simulink model "ModeleRobot"  (Simulink 7.4)
settings: Solver=FixedStepDiscrete  StartTime=0.0  StopTime=Inf  FixedStep=Te  RelTol=1e-3
libraries: simulink x10
CloseFcn:
  | rtwprivate ssgencode ModelCloseRequest ModeleRobot
settings Model: Creator=Admin  LastModifiedBy=Admin
settings DataIOCC: LimitDataPoints=off  SaveFormat=StructureWithTime
settings OptimizationCC: UseIntDivNetSlope=on  PassReuseOutputArgsAs=Individual arguments  ZeroExternalMemoryAtStartup=off  ZeroInternalMemoryAtStartup=off  EfficientFloat2IntCast=on  OptimizeModelRefInitCode=on  LifeSpan=Inf
settings DebuggingCC: SaveWithParameterizedLinksMsg=none  SignalResolutionControl=TryResolveAllWithWarning  MultiTaskDSMMsg=warning  MultiTaskCondExecSysMsg=none
settings HardwareCC: ProdIntDivRoundTo=Zero  ProdEndianess=LittleEndian  ProdHWDeviceType=Generic->32-bit x86 compatible
settings SFSimCC: SFSimEnableDebug=off  SFSimOverflowDetection=off  SFSimEcho=off  SimIntegrity=off  SimBuildMode=sf_nonincremental_build
settings RTWCC: SystemTargetFile=ert.tlc  GenCodeOnly=on  GenerateMakefile=off  TemplateMakefile=ert_default_tmf  PostCodeGenCommand=packNGo(buildInfo);  Description=Real-Time Workshop Embedded Coder  ProcessScript=ert_make_rtw_hook  IncludeERTFirstTime=on  RTWCompilerOptimization=On  CheckMdlBeforeBuild=Warning
settings CodeAppCC: IgnoreCustomStorageClasses=off
settings ERTTargetCC: UtilityFuncGeneration=Shared location  MultiwordLength=2048  IncludeMdlTerminateFcn=off  SuppressErrorStatus=on  SupportNonFinite=off  ERTCustomFileTemplate=example_file_process.tlc  GlobalDataDefinition=InSourceFile  GlobalDataReference=InSourceFile  ConvertIfToSwitch=off

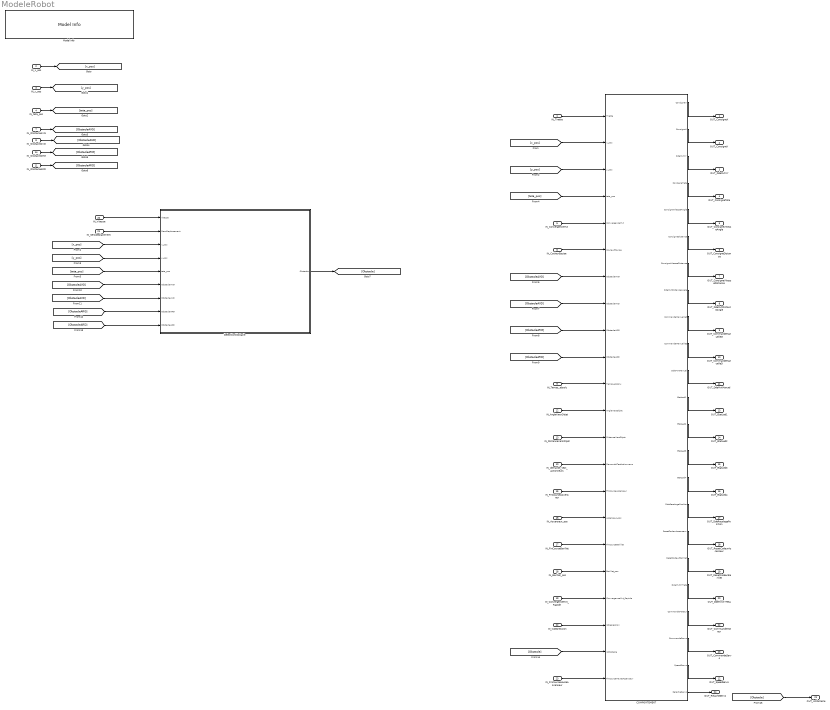
== system ModeleRobot ==
  IN_Tirette : Inport  OutDataType=sfix(16)  OutScaling=2^0
  IN_x_pos : Inport  Port=2  OutDataType=sfix(16)  OutScaling=2^0
  IN_y_pos : Inport  Port=3  OutDataType=sfix(16)  OutScaling=2^0
  IN_teta_pos : Inport  Port=4  OutDataType=sfix(16)  OutScaling=2^0
  IN_ConvergenceMvt : Inport  Port=5  OutDataType=sfix(16)  OutScaling=2^0
  IN_CouleurEquipe : Inport  Port=6  OutDataType=sfix(16)  OutScaling=2^0
  IN_ObstacleAVG : Inport  Port=7  OutDataType=sfix(16)  OutScaling=2^0
  IN_ObstacleAVD : Inport  Port=8  OutDataType=sfix(16)  OutScaling=2^0
  IN_Temps_absolu : Inport  Port=9  OutDataType=sfix(16)  OutScaling=2^0
  IN_demande_test_actionneurs : Inport  Port=10  OutDataType=sfix(16)  OutScaling=2^0
  IN_ObstacleARD : Inport  Port=11  OutDataType=sfix(16)  OutScaling=2^0
  IN_AngleVersObjet : Inport  Port=12  OutDataType=sfix(16)  OutScaling=2^0
  IN_DistanceVersObjet : Inport  Port=13  OutDataType=sfix(16)  OutScaling=2^0
  IN_ObstacleARG : Inport  Port=14  OutDataType=sfix(16)  OutScaling=2^0
  IN_FinCourseAscenseur : Inport  Port=15  OutDataType=sfix(16)  OutScaling=2^0
  IN_Ascenseur_pos : Inport  Port=16  OutDataType=sfix(16)  OutScaling=2^0
  IN_FinCourseBarillet : Inport  Port=17  OutDataType=sfix(16)  OutScaling=2^0
  IN_Barillet_pos : Inport  Port=18  OutDataType=sfix(16)  OutScaling=2^0
  IN_ConvergenceMvt_Rapide : Inport  Port=19  OutDataType=sfix(16)  OutScaling=2^0
  IN_Vitesse : Inport  Port=20  OutDataType=sfix(16)  OutScaling=2^0
  IN_SensDeplacement : Inport  Port=21  OutDataType=sfix(16)  OutScaling=2^0
  IN_isDepression : Inport  Port=22  OutDataType=sfix(16)  OutScaling=2^0
  IN_FinCourseHauteAscenseur : Inport  Port=23  OutDataType=sfix(16)  OutScaling=2^0
  COMPORTEMENT : Stateflow chart
  DetectionObstacle : Subsystem
  Model Info : simulink/Model-Wide Utilities/Model Info  SystemSampleTime=-1  InitialBlockCM=None  BlockCM=None  Frame=on  DisplayStringWithTags=|  HorizontalTextAlignment=Left  LeftAlignmentValue=0.02  SourceBlockDiagram=ModeleRobot  TagMaxNumber=20
      | Description du comportement d'un robot
      | Objectif du robot :
  OUT_ConsigneX : Outport  OutDataType=sfix(16)  OutScaling=2^0
  OUT_ConsigneY : Outport  Port=2  OutDataType=sfix(16)  OutScaling=2^0
  OUT_DdeMvtXY : Outport  Port=3  OutDataType=sfix(16)  OutScaling=2^0
  OUT_ConsigneTeta : Outport  Port=4  OutDataType=sfix(16)  OutScaling=2^0
  OUT_ConsigneVitesseAngle : Outport  Port=5  OutDataType=sfix(16)  OutScaling=2^0
  OUT_ConsigneDistance : Outport  Port=6  OutDataType=sfix(16)  OutScaling=2^0
  OUT_ConsigneVitesseDistance : Outport  Port=7  OutDataType=sfix(16)  OutScaling=2^0
  OUT_DdeMvtDistanceAngle : Outport  Port=8  OutDataType=sfix(16)  OutScaling=2^0
  OUT_CommandeManuelleG : Outport  Port=9  OutDataType=sfix(16)  OutScaling=2^0
  OUT_CommandeManuelleD : Outport  Port=10  OutDataType=sfix(16)  OutScaling=2^0
  OUT_DdeMvtManuel : Outport  Port=11  OutDataType=sfix(16)  OutScaling=2^0
  OUT_SpeedServo : Outport  Port=12  OutDataType=sfix(16)  OutScaling=2^0
  OUT_EtatLed1 : Outport  Port=13  OutDataType=sfix(16)  OutScaling=2^0
  OUT_EtatLed2 : Outport  Port=14  OutDataType=sfix(16)  OutScaling=2^0
  OUT_EtatLed3 : Outport  Port=15  OutDataType=sfix(16)  OutScaling=2^0
  OUT_EtatLed4 : Outport  Port=16  OutDataType=sfix(16)  OutScaling=2^0
  OUT_DdeRecalagePosition : Outport  Port=17  OutDataType=sfix(16)  OutScaling=2^0
  OUT_ResetCodeurAscenseur : Outport  Port=18  OutDataType=sfix(16)  OutScaling=2^0
  OUT_ResetCodeurBarillet : Outport  Port=19  OutDataType=sfix(16)  OutScaling=2^0
  OUT_DdeMvtXYTeta : Outport  Port=20  OutDataType=sfix(16)  OutScaling=2^0
  OUT_isObstacle : Outport  Port=21  OutDataType=sfix(16)  OutScaling=2^0
  OUT_CommandeMoteur : Outport  Port=22  OutDataType=sfix(16)  OutScaling=2^0
  OUT_CommandeServo : Outport  Port=23  OutDataType=sfix(16)  OutScaling=2^0
  OUT_RelacheServo : Outport  Port=24  OutDataType=sfix(16)  OutScaling=2^0
  wires:
  COMPORTEMENT/1(ConsigneX) -> OUT_ConsigneX/1
  COMPORTEMENT/2(ConsigneY) -> OUT_ConsigneY/1
  IN_Temps_absolu/1 -> COMPORTEMENT/11(Temps_absolu)
  IN_ConvergenceMvt/1 -> COMPORTEMENT/5(ConvergenceMvt)
  IN_CouleurEquipe/1 -> COMPORTEMENT/6(CouleurEquipe)
  IN_Tirette/1 -> COMPORTEMENT/1(Tirette)
  IN_demande_test_actionneurs/1 -> COMPORTEMENT/14(DemandeTestActionneurs)
  IN_AngleVersObjet/1 -> COMPORTEMENT/12(AngleVersObjet)
  IN_DistanceVersObjet/1 -> COMPORTEMENT/13(DistanceVersObjet)
  COMPORTEMENT/3(DdeMvtXY) -> OUT_DdeMvtXY/1
  COMPORTEMENT/4(ConsigneTeta) -> OUT_ConsigneTeta/1
  COMPORTEMENT/5(ConsigneVitesseAngle) -> OUT_ConsigneVitesseAngle/1
  COMPORTEMENT/6(ConsigneDistance) -> OUT_ConsigneDistance/1
  COMPORTEMENT/7(ConsigneVitesseDistance) -> OUT_ConsigneVitesseDistance/1
  COMPORTEMENT/8(DdeMvtDistanceAngle) -> OUT_DdeMvtDistanceAngle/1
  COMPORTEMENT/9(CommandeManuelleG) -> OUT_CommandeManuelleG/1
  COMPORTEMENT/10(CommandeManuelleD) -> OUT_CommandeManuelleD/1
  COMPORTEMENT/11(DdeMvtManuel) -> OUT_DdeMvtManuel/1
  COMPORTEMENT/22(SpeedServo) -> OUT_SpeedServo/1
  COMPORTEMENT/12(EtatLed1) -> OUT_EtatLed1/1
  COMPORTEMENT/13(EtatLed2) -> OUT_EtatLed2/1
  COMPORTEMENT/14(EtatLed3) -> OUT_EtatLed3/1
  COMPORTEMENT/15(EtatLed4) -> OUT_EtatLed4/1
  COMPORTEMENT/16(DdeRecalagePosition) -> OUT_DdeRecalagePosition/1
  COMPORTEMENT/17(ResetCodeurAscenseur) -> OUT_ResetCodeurAscenseur/1
  COMPORTEMENT/18(ResetCodeurBarillet) -> OUT_ResetCodeurBarillet/1
  [x_pos] -> COMPORTEMENT/2(x_pos)
  [y_pos] -> COMPORTEMENT/3(y_pos)
  [teta_pos] -> COMPORTEMENT/4(teta_pos)
  IN_Vitesse/1 -> DetectionObstacle/1(Vitesse)
  IN_SensDeplacement/1 -> DetectionObstacle/2(SensDeplacement)
  [x_pos] -> DetectionObstacle/3(x_pos)
  [y_pos] -> DetectionObstacle/4(y_pos)
  [teta_pos] -> DetectionObstacle/5(teta_pos)
  IN_x_pos/1 -> [x_pos]
  IN_y_pos/1 -> [y_pos]
  IN_teta_pos/1 -> [teta_pos]
  COMPORTEMENT/19(DdeMvtXYTeta) -> OUT_DdeMvtXYTeta/1
  IN_ObstacleAVG/1 -> [ObstacleAVG]
  IN_ObstacleAVD/1 -> [ObstacleAVD]
  IN_ObstacleARG/1 -> [ObstacleARG]
  IN_ObstacleARD/1 -> [ObstacleARD]
  [ObstacleAVG] -> COMPORTEMENT/7(ObstacleAVG)
  [ObstacleAVD] -> COMPORTEMENT/8(ObstacleAVD)
  [ObstacleARG] -> COMPORTEMENT/9(ObstacleARG)
  [ObstacleARD] -> COMPORTEMENT/10(ObstacleARD)
  [ObstacleAVG] -> DetectionObstacle/6(ObstacleAVG)
  [ObstacleAVD] -> DetectionObstacle/7(ObstacleAVD)
  [ObstacleARG] -> DetectionObstacle/8(ObstacleARG)
  [ObstacleARD] -> DetectionObstacle/9(ObstacleARD)
  DetectionObstacle/1(Obstacle) -> [Obstacle]
  IN_FinCourseAscenseur/1 -> COMPORTEMENT/15(FinCourseAscenseur)
  [Obstacle] -> COMPORTEMENT/21(isObstacle)
  IN_FinCourseHauteAscenseur/1 -> COMPORTEMENT/22(FinCourseHauteAscenseur)
  IN_Ascenseur_pos/1 -> COMPORTEMENT/16(Ascenseur_pos)
  IN_FinCourseBarillet/1 -> COMPORTEMENT/17(FinCourseBarillet)
  IN_Barillet_pos/1 -> COMPORTEMENT/18(Barillet_pos)
  IN_ConvergenceMvt_Rapide/1 -> COMPORTEMENT/19(ConvergenceMvt_Rapide)
  IN_isDepression/1 -> COMPORTEMENT/20(isDepression)
  [Obstacle] -> OUT_isObstacle/1
  COMPORTEMENT/21(CommandeServo) -> OUT_CommandeServo/1
  COMPORTEMENT/20(CommandeMoteur) -> OUT_CommandeMoteur/1
  COMPORTEMENT/23(RelacheServo) -> OUT_RelacheServo/1

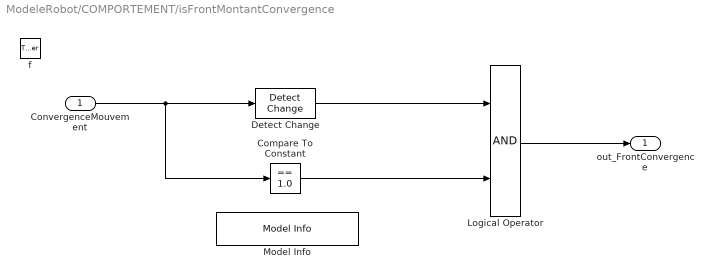
== system ModeleRobot/COMPORTEMENT/isFrontMontantConvergence ==
  ConvergenceMouvement : Inport
  f : TriggerPort  TriggerType=function-call
      settings: CopyFcn=set_param(gcbh,'PreDeleteFcn','')  PreDeleteFcn=Stateflow.SLINSF.SimulinkMan.unsafePredeleteFcn
  Compare To Constant : simulink/Logic and Bit Operations/Compare To Constant  SystemSampleTime=-1  relop===  const=1.0  LogicOutDataTypeMode=uint8
  Detect Change : simulink/Logic and Bit Operations/Detect Change  SystemSampleTime=-1  vinit=0
  Logical Operator : Logic  AllPortsSameDT=off  OutDataTypeMode=boolean  LogicDataType=fixdt(0, 8)  OutDataTypeStr=boolean
  Model Info : simulink/Model-Wide Utilities/Model Info  SystemSampleTime=-1  InitialBlockCM=None  BlockCM=None  Frame=off  DisplayStringWithTags="\"1\" = mouvement terminé"  HorizontalTextAlignment=Center  LeftAlignmentValue=0.5  SourceBlockDiagram=ModeleRobot  TagMaxNumber=20
  out_FrontConvergence : Outport
  wires:
  ConvergenceMouvement/1 -> Detect Change/1, Compare To Constant/1
  Detect Change/1 -> Logical Operator/1
  Compare To Constant/1 -> Logical Operator/2
  Logical Operator/1 -> out_FrontConvergence/1

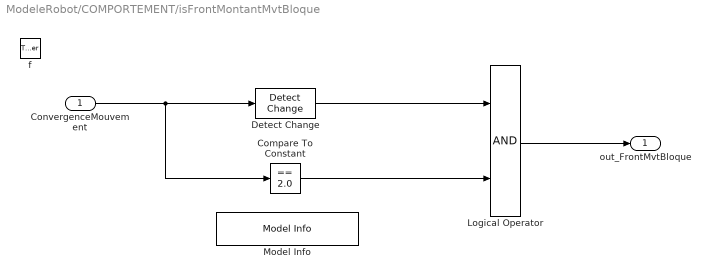
== system ModeleRobot/COMPORTEMENT/isFrontMontantMvtBloque ==
  ConvergenceMouvement : Inport
  f : TriggerPort  TriggerType=function-call
      settings: CopyFcn=set_param(gcbh,'PreDeleteFcn','')  PreDeleteFcn=Stateflow.SLINSF.SimulinkMan.unsafePredeleteFcn
  Compare To Constant : simulink/Logic and Bit Operations/Compare To Constant  SystemSampleTime=-1  relop===  const=2.0  LogicOutDataTypeMode=uint8
  Detect Change : simulink/Logic and Bit Operations/Detect Change  SystemSampleTime=-1  vinit=0
  Logical Operator : Logic  AllPortsSameDT=off  OutDataTypeMode=boolean  LogicDataType=fixdt(0, 8)  OutDataTypeStr=boolean
  Model Info : simulink/Model-Wide Utilities/Model Info  SystemSampleTime=-1  InitialBlockCM=None  BlockCM=None  Frame=off  DisplayStringWithTags="\"2\" = mouvement bloqué"  HorizontalTextAlignment=Center  LeftAlignmentValue=0.5  SourceBlockDiagram=ModeleRobot  TagMaxNumber=20
  out_FrontMvtBloque : Outport
  wires:
  ConvergenceMouvement/1 -> Detect Change/1, Compare To Constant/1
  Detect Change/1 -> Logical Operator/1
  Compare To Constant/1 -> Logical Operator/2
  Logical Operator/1 -> out_FrontMvtBloque/1

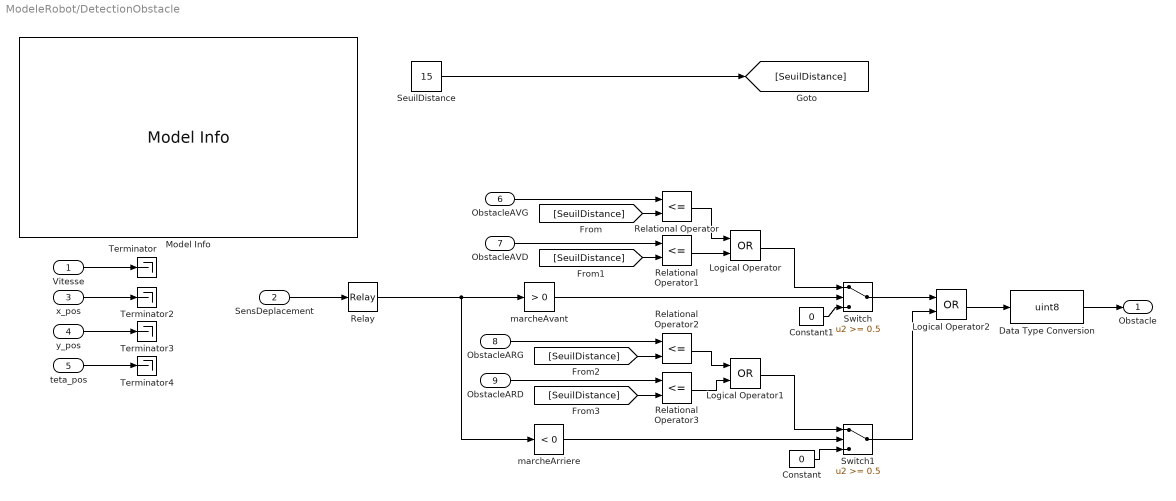
== system ModeleRobot/DetectionObstacle ==
  Vitesse : Inport  OutDataType=fixdt(1, 16)  OutScaling=2^0
  SensDeplacement : Inport  Port=2  OutDataType=fixdt(1, 16)  OutScaling=2^0
  x_pos : Inport  Port=3  OutDataType=fixdt(1, 16)  OutScaling=2^0
  y_pos : Inport  Port=4  OutDataType=fixdt(1, 16)  OutScaling=2^0
  teta_pos : Inport  Port=5  OutDataType=fixdt(1, 16)  OutScaling=2^0
  ObstacleAVG : Inport  Port=6  OutDataType=fixdt(1, 16)  OutScaling=2^0
  ObstacleAVD : Inport  Port=7  OutDataType=fixdt(1, 16)  OutScaling=2^0
  ObstacleARG : Inport  Port=8  OutDataType=fixdt(1, 16)  OutScaling=2^0
  ObstacleARD : Inport  Port=9  OutDataType=fixdt(1, 16)  OutScaling=2^0
  Constant : Constant  Value=0  OutDataType=fixdt(1, 16)  OutScaling=2^0
  Constant1 : Constant  Value=0  OutDataType=fixdt(1, 16)  OutScaling=2^0
  Data Type Conversion : DataTypeConversion  OutDataTypeMode=uint8  OutDataType=fixdt(1, 16)  OutScaling=2^0  OutDataTypeStr=uint8
  Logical Operator : Logic  Operator=OR  AllPortsSameDT=off  OutDataTypeMode=boolean  LogicDataType=fixdt(0, 8)  OutDataTypeStr=boolean
  Logical Operator1 : Logic  Operator=OR  AllPortsSameDT=off  OutDataTypeMode=boolean  LogicDataType=fixdt(0, 8)  OutDataTypeStr=boolean
  Logical Operator2 : Logic  Operator=OR  AllPortsSameDT=off  OutDataTypeMode=boolean  LogicDataType=fixdt(0, 8)  OutDataTypeStr=boolean
  Model Info : simulink/Model-Wide Utilities/Model Info  SystemSampleTime=-1  InitialBlockCM=None  BlockCM=None  Frame=on  DisplayStringWithTags=|  HorizontalTextAlignment=Left  LeftAlignmentValue=0.02  SourceBlockDiagram=ModeleRobot  TagMaxNumber=20
      | Description de la détection d'obstacle
      | Obstacle :
      | Suivant le sens de la marche on active la détection par capteur US (donne une distance). Fonction d'un seuil de distance on tilte sur la présence d'un obstacle. On synthétise les détection arrière et avant pour avoir une seule info de détection d'obstacle pour la stratégie.
      | 
      | TODO:
      | * faire varier le seuil de détection en fonction de la vitesse.
      | * utiliser la position et l'orientation du robot pour discriminer un élément du terrain.
  Relational Operator{,1..3} (4 alike) : RelationalOperator  Operator=<=  LogicOutDataTypeMode=boolean  LogicDataType=fixdt(0, 8)  OutDataTypeStr=boolean
  Relay : Relay  OnSwitchValue=1  OffSwitchValue=-1  OffOutputValue=-1  OutDataType=fixdt(1, 16)  OutScaling=2^0
  SeuilDistance : Constant  Value=15  OutDataType=fixdt(1, 16)  OutScaling=2^0
  Switch : Switch  Threshold=0.5  OutDataType=fixdt(1, 16)  OutScaling=2^0
  Switch1 : Switch  Threshold=0.5  OutDataType=fixdt(1, 16)  OutScaling=2^0
  Terminator{,2..4} (4 alike) : Terminator
  marcheArriere : simulink/Logic and Bit Operations/Compare To Zero  SystemSampleTime=-1  relop=<  LogicOutDataTypeMode=uint8
  marcheAvant : simulink/Logic and Bit Operations/Compare To Zero  SystemSampleTime=-1  relop=>  LogicOutDataTypeMode=uint8
  Obstacle : Outport  OutDataType=fixdt(1, 16)  OutScaling=2^0
  wires:
  Vitesse/1 -> Terminator/1
  SensDeplacement/1 -> Relay/1
  x_pos/1 -> Terminator2/1
  y_pos/1 -> Terminator3/1
  teta_pos/1 -> Terminator4/1
  marcheAvant/1 -> Switch/2
  Relational Operator1/1 -> Logical Operator/2
  ObstacleARD/1 -> Relational Operator3/1
  marcheArriere/1 -> Switch1/2
  Relational Operator2/1 -> Logical Operator1/1
  Constant/1 -> Switch1/3
  Switch/1 -> Logical Operator2/1
  Switch1/1 -> Logical Operator2/2
  Logical Operator2/1 -> Data Type Conversion/1
  Relational Operator/1 -> Logical Operator/1
  ObstacleAVG/1 -> Relational Operator/1
  ObstacleAVD/1 -> Relational Operator1/1
  ObstacleARG/1 -> Relational Operator2/1
  SeuilDistance/1 -> [SeuilDistance]
  [SeuilDistance] -> Relational Operator/2
  [SeuilDistance] -> Relational Operator3/2
  [SeuilDistance] -> Relational Operator2/2
  [SeuilDistance] -> Relational Operator1/2
  Constant1/1 -> Switch/3
  Relational Operator3/1 -> Logical Operator1/2
  Logical Operator1/1 -> Switch1/1
  Logical Operator/1 -> Switch/1
  Data Type Conversion/1 -> Obstacle/1
  Relay/1 -> marcheAvant/1, marcheArriere/1

== stateflow chart COMPORTEMENT ==
  state COMPORTEMENT_ROBOT [parallel]
    settings: executionOrder=1
    state ATTENTE_TIRETTE/
      state ACTIONNEURS_REPOS/ [parallel]
        settings: executionOrder=1
        state REPOS_SERVOS/
          entry :
          //on ne bouge pas en attendant le depart
          Mouvement_Manuel(0, 0);
          setPWM(MOTEUR_ASCENSEUR,0);
          setPWM(MOTEUR_DISTRIBUTEUR,0);
          setPWM(MOTEUR_NON_DEFINI,0);
          setPWM(MOTEUR_SOUFFLEUR,0);
          //meme si la vitesse n'est pas utilise, on l'initialise pour les servos
          setServoSpeed(SERVO_PINCE_G,MAX_SPEED_SERVOS);
          setServoSpeed(SERVO_PINCE_D,MAX_SPEED_SERVOS);
          setServoSpeed(SERVO_CENTREUR_G,MAX_SPEED_SERVOS);
          setServoSpeed(SERVO_CENTREUR_D,MAX_SPEED_SERVOS);
          //de meme pour le maintient ou non des servos on initialise
          setServoRelache(SERVO_PINCE_G,0);
          setServoRelache(SERVO_PINCE_D,0);
          setServoRelache(SERVO_CENTREUR_G,1);
          setServoRelache(SERVO_CENTREUR_D,1);
          //on ecarte les pinces pour qu'elles soient bien dans le robot
          setServo(SERVO_PINCE_G,SERVO_PINCE_G_OUVERT);
          setServo(SERVO_PINCE_D,SERVO_PINCE_D_OUVERT);
          //l'inverse pour les centreurs
          setServo(SERVO_CENTREUR_G,SERVO_CENTREUR_G_FERME);
          setServo(SERVO_CENTREUR_D,SERVO_CENTREUR_D_FERME);
          //on lance le timer pour laisser un petit temps aux actions precedentes
          TempoInit=0;
          during:
          TempoInit++;
        state APPRENTISSAGE_KMAR_01/
          entry:
          //les pinces sont rangees on peut descendre l'ascenseur
          setPWM(MOTEUR_ASCENSEUR,-60);
          //meme si on a un capteur de fin de course, par securite on met une tempo
          TempoInit=0;
          during:
          TempoInit++;
        state APPRENTISSAGE_KMAR_02/
          entry:
          //on est en butee on arrete immediatement l'ascenseur
          setPWM(MOTEUR_ASCENSEUR,0);
          //On fait le reset du codeur ascenseur
          ResetCodeurAscenseur=1;
          TempoInit=0;
          during:
          TempoInit++;
        state FIN_REPOS_ACTIONNEUR/
          entry:
          //on arrete l'ascenseur
          setPWM(MOTEUR_ASCENSEUR,0);
        state APPRENTISSAGE_KMAR_03/
          entry:
          //on remonte l'ascenseur jusqu'a la position d'un feu en haut de la torche
          setPWM(MOTEUR_ASCENSEUR,60);
          //On relache le reset du codeur ascenseur
          ResetCodeurAscenseur=0;
          //meme si on a un apprentissage des positions par securite on met une tempo
          TempoInit=0;
          during:
          TempoInit++;
        (default) -> REPOS_SERVOS
        REPOS_SERVOS -> APPRENTISSAGE_KMAR_01 : [TempoInit>(2/Te)]
        APPRENTISSAGE_KMAR_03 -> FIN_REPOS_ACTIONNEUR : [(Ascenseur_pos>=KMAR_POSITION_DEPART) || (TempoInit>(4/Te))]
        APPRENTISSAGE_KMAR_01 -> APPRENTISSAGE_KMAR_02 : [(FinCourseAscenseur==1) || (TempoInit>(5/Te))]
        APPRENTISSAGE_KMAR_02 -> APPRENTISSAGE_KMAR_03 : [TempoInit>(1/Te)]
      state CHOIX_EQUIPE/ [parallel]
        exit :
        CouleurEquipe_memo = CouleurEquipe;
        settings: executionOrder=2
        state EQUIPE_2/
          entry :
          EtatLed1 = 0;
          EtatLed2 = 1;
          invMouv=1;
        state EQUIPE_1/
          entry :
          EtatLed1 = 1;
          EtatLed2 = 0;
          invMouv=-1;
        (default) -> EQUIPE_1
        EQUIPE_1 -> EQUIPE_2 : [CouleurEquipe == EQUIPE_JAUNE]
        EQUIPE_2 -> EQUIPE_1 : [CouleurEquipe == EQUIPE_VERTE]
      state RECALAGE/ [parallel]
        //TODO: a faire si on veut respecter le terrain
        entry:
        TempoMot=0;
        during:
        TempoMot++;
        settings: executionOrder=3
      state TESTS_ACTIONNEUR/ [parallel]
        entry:
        TempoTestActionneurs=0;
        during :
        TempoTestActionneurs++;
        settings: executionOrder=4
        state TEST_ACT_FIN/
          entry:
          TempoTestActionneurs = 0;
          test_actionneurs_en_cours=0;
        state INIT/
          entry:
          test_actionneurs_en_cours=0;
        state TEST_ACT_1/
          entry:
          TempoTestActionneurs = 0;
          setServo(SERVO_PINCE_G, SERVO_PINCE_G_FERME);
        state TEST_ACT_3/
          entry:
          TempoTestActionneurs = 0;
          setServo(SERVO_PINCE_D, SERVO_PINCE_D_OUVERT);
        state INIT1/
          entry:
          test_actionneurs_en_cours=1;
          TempoTestActionneurs = 0;
        state TEST_ACT_2/
          entry:
          TempoTestActionneurs = 0;
          setServo(SERVO_PINCE_G, SERVO_PINCE_G_OUVERT);
          setServo(SERVO_PINCE_D, SERVO_PINCE_D_FERME);
        (junction 128) -> INIT1 : [DemandeTestActionneurs != 0]
        TEST_ACT_FIN -> (junction 128)
        (default) -> INIT
        INIT -> (junction 128)
        INIT1 -> TEST_ACT_1 : [TempoTestActionneurs > (2/Te)]
        TEST_ACT_1 -> TEST_ACT_2 : [TempoTestActionneurs > (2/Te)]
        TEST_ACT_3 -> TEST_ACT_FIN : [TempoTestActionneurs > (2/Te)]
        TEST_ACT_2 -> TEST_ACT_3 : [TempoTestActionneurs > (2/Te)]
    state FIN_MATCH/
      state FIN_MATCH_01/
        entry:
        Mouvement_Manuel(0, 0);
        setServo(SERVO_PINCE_G,SERVO_PINCE_G_OUVERT);
        setServo(SERVO_PINCE_D,SERVO_PINCE_D_OUVERT);
        CommandeLEDS_RVBO(1, 1, 1, 1);
      state FIN_MATCH_02/
        entry:
        //chenillard de led
        CommandeLEDS_RVBO(1, 0, 0, 0);
        TempoImage=0;
        during:
        TempoImage++;
      state FIN_MATCH_04/
        entry:
        //chenillard de led
        CommandeLEDS_RVBO(0, 0, 1, 0);
        TempoImage=0;
        during:
        TempoImage++;
      state FIN_MATCH_05/
        entry:
        //chenillard de led
        CommandeLEDS_RVBO(0, 0, 0, 1);
        TempoImage=0;
        during:
        TempoImage++;
      state FIN_MATCH_03/
        entry:
        //chenillard de led
        CommandeLEDS_RVBO(0, 1, 0, 0);
        TempoImage=0;
        during:
        TempoImage++;
      FIN_MATCH_05 -> FIN_MATCH_02 : [(TempoImage>(1/Te))]
      FIN_MATCH_01 -> FIN_MATCH_02
      (default) -> FIN_MATCH_01
      FIN_MATCH_02 -> FIN_MATCH_03 : [(TempoImage>(1/Te))]
      FIN_MATCH_03 -> FIN_MATCH_04 : [(TempoImage>(1/Te))]
      FIN_MATCH_04 -> FIN_MATCH_05 : [(TempoImage>(1/Te))]
    state MATCH/
      state STRATEGIE/ [parallel]
        settings: executionOrder=2
        state STRATEGIE1
          (history)
          state INIT_STRATEGIE/
            entry :
            ConsigneVitesseAngle = 3; // [rad/sec]
            ConsigneVitesseDistance = 40; //[cm/sec]
            AutoriseDetectionObstacle_AV = 0;
            AutoriseDetectionObstacle_AR = 0;
            finHomologation=0;
            ElementPiege_AV = 0;
            ElementPiege_AR = 0;
            //pour 2015 on part en marche arrière
            setPosition(0,0,PI);
          state DEMO/
            entry:
            TempoMot=0;
            DistanceParcourue=0;DistanceParcourue2=0;
            x_old=0;y_old=0;   x_old2=0;y_old2=0;
            x_temp=0;y_temp=0;
            cmptServos=0;
            inhibeObstacle=0;
            during:
            TempoMot++;
            //CommandeLEDS_RVBO(ObstacleARG,ObstacleARD, ObstacleAVG,ObstacleAVD);vv
            (history)
            state ACTION_12
              entry:
              Mouvement_XYTeta(-3.00,65.00,-1.5700); /*en position pour ramasser les popcorn*/
            state ACTION_10
              entry:
              Mouvement_XYTeta(27.00,65.00,-1.5700); /*j ai les premiers popcorn je degage*/
            state ACTION_14
              entry:
              Mouvement_XYTeta(-3.00,65.00,-1.5700); /*j ai tous les popcorn je degage*/
            state ACTION_2
              entry:
              Mouvement_XYTeta(46.00,61.00,1.5700); /*ramassage d un spot*/
              inhibeObstacle=1;
            state ACTION_6
              entry:
              Mouvement_XYTeta(27.00,65.00,-1.5700); /*en position pour ramasser les popcorn*/
            state ACTION_4
              entry:
              Mouvement_XYTeta(46.00,68.00,1.5700); /*ramassage d un deuxieme spot*/
            state ACTION_8
              entry:
              Mouvement_XYTeta(27.00,76.00,-1.5700); /*accostage distri 1*/
            state ACTION_0
              entry:
              Mouvement_XYTeta(46.00,0.00,0.0000);
            state ACTION_18
              entry:
              Mouvement_XYTeta(46.00,0.00,-1.5700);
              finHomologation=1;
            state ACTION_16
              entry:
              Mouvement_XYTeta(-3.00,76,-1.5700); /*accostage distri 1*/
            state ACTION_HOMOLO_0
              entry:
              setPWM(MOTEUR_ASCENSEUR,0);
              TempoMot=0;
            state ACTION_HOMOLO_2
              entry:
              //on fait une diagonale pour pousser le deuxieme spots dans la zone de construction
              Mouvement_XYTeta(85,-72*invMouv,-0.99*invMouv);
              exit:
              setServo(SERVO_PINCE_G,SERVO_PINCE_G_OUVERT);
              setServo(SERVO_PINCE_D,SERVO_PINCE_D_OUVERT);
            state ACTION_HOMOLO_4
              entry:
              Mouvement_XYTeta(38,0,0);
            state ACTION_HOMOLO_5
              entry:
              Mouvement_XYTeta(2,0,0);
            state ACTION_HOMOLO_01
              entry:
              //on prend la balle de tennis
              setServo(SERVO_PINCE_G,SERVO_PINCE_G_FERME);
              setServo(SERVO_PINCE_D,SERVO_PINCE_D_FERME);
              //tempo
              TempoMot=0;
            state ACTION_HOMOLO_02
              entry:
              //on monte l'ascenseur pour etre au dessus d'un spot
              setPWM(MOTEUR_ASCENSEUR,60);
              //tempo
              TempoMot=0;
            state ACTION_HOMOLO_6
              entry:
              //on se dirige vers le 1er spot
              Mouvement_XYTeta(60,-27*invMouv,-1.06*invMouv);
            state ACTION_HOMOLO_7
              entry:
              inhibeObstacle=0;
              //on se tourne vers les spots
              Mouvement_Angle(-0.99*invMouv);
            state ACTION_HOMOLO_8
              entry:
              //on relache la balle
              //TODO: rechercher une position intermédiaire servo pour retenir balle + spot
              setServo(SERVO_PINCE_G,SERVO_PINCE_G_ENTRE_OUVERT);
              setServo(SERVO_PINCE_D,SERVO_PINCE_D_ENTRE_OUVERT);
              TempoMot=0;
            state ACTION_HOMOLO_9
              entry:
              //on accoste le distributeur à 10 cm
              Mouvement_XYTeta(36,65,-1.57);
            state ACTION_HOMOLO_10
              entry:
              inhibeObstacle=0;
              //on se tourne vers le distributeur en lui presentant l'arriere du robot
              Mouvement_Angle(-1.57);
            state ACTION_HOMOLO_11
              entry:
              //pas de robot possible dans ce coin, on inhibe la detection d'obstacle
              Mouvement_XYTeta(36,75,-1.57);
            state ACTION_HOMOLO_12
              entry:
              //on sort les recolteurs et on leur laisse 1sec
              TempoMot=0;
              setServo(SERVO_RECOLTEURS,SERVO_RECOLTEURS_OUVERT);
            state ACTION_HOMOLO_13
              entry:
              //on souffle pendant 2 secondes
              TempoMot=0;
              setPWM(MOTEUR_SOUFFLEUR,100);
            state ACTION_HOMOLO_14
              entry:
              //on arrete de souffler et on rentre les recolteurs
              setPWM(MOTEUR_SOUFFLEUR,0);
              setServo(SERVO_RECOLTEURS,SERVO_RECOLTEURS_FERME);
            state ACTION_HOMOLO_03
              entry:
              //on sort de la zone de départ
              //on a mis une tempo pour minibot et desactiver la detection d'obstacle
              //pour le defoncer s'il merde, a priori l'action avec la balle dure juste ce qu'il faut (à potarder)
              inhibeObstacle=1;
              Mouvement_XYTeta(38,0,PI);
            ACTION_8 -> ACTION_10 : [isFinMouvement(5/Te)]
            ACTION_0 -> ACTION_2 : [isFinMouvement(5/Te)]
            ACTION_4 -> ACTION_6 : [isFinMouvement(5/Te)]
            ACTION_2 -> ACTION_4 : [isFinMouvement(5/Te)]
            ACTION_10 -> ACTION_12 : [isFinMouvement(5/Te)]
            ACTION_6 -> ACTION_8 : [isFinMouvement(5/Te)]
            ACTION_HOMOLO_5 -> ACTION_0 : [(isFinMouvement(5/Te) && (JUST_HOMOLO==0))]
            ACTION_12 -> ACTION_14 : [isFinMouvement(5/Te)]
            ACTION_16 -> ACTION_18 : [isFinMouvement(5/Te)]
            ACTION_14 -> ACTION_16 : [isFinMouvement(5/Te)]
            (default) -> ACTION_HOMOLO_01
            ACTION_HOMOLO_6 -> ACTION_HOMOLO_8 : [isFinMouvement(3/Te)]
            ACTION_HOMOLO_2 -> ACTION_HOMOLO_4 : [isFinMouvement(5/Te)]
            ACTION_HOMOLO_4 -> ACTION_HOMOLO_5 : [isFinMouvement(5/Te)]
            ACTION_HOMOLO_02 -> ACTION_HOMOLO_0 : [(Ascenseur_pos>=KMAR_POSITION_AU_DESSUS_SPOT_SANS_SPOT) || (TempoMot>(4/Te))]
            ACTION_HOMOLO_01 -> ACTION_HOMOLO_02 : [TempoMot>(1/Te)]
            ACTION_HOMOLO_7 -> ACTION_HOMOLO_6 : [isFinMouvement(2/Te)]
            ACTION_HOMOLO_0 -> ACTION_HOMOLO_03 : [TempoMot>(1/Te)]
            ACTION_HOMOLO_8 -> ACTION_HOMOLO_2 : [TempoMot>(2/Te)]
            ACTION_HOMOLO_10 -> ACTION_HOMOLO_9 : [isFinMouvement(5/Te)]
            ACTION_HOMOLO_9 -> ACTION_HOMOLO_11 : [isFinMouvement(5/Te)]
            ACTION_HOMOLO_11 -> ACTION_HOMOLO_12 : [isFinMouvement(5/Te)]
            ACTION_HOMOLO_12 -> ACTION_HOMOLO_13 : [TempoMot>(1/Te)]
            ACTION_HOMOLO_13 -> ACTION_HOMOLO_14 : [TempoMot>(2/Te)]
            ACTION_HOMOLO_03 -> ACTION_HOMOLO_7 : [isFinMouvement(3/Te)]
          (default) -> INIT_STRATEGIE
          INIT_STRATEGIE -> DEMO : [DureeMatch > (0.5/Te)]
        state EVITEMENT/
          entry :
          EvitementEnCours  = 1;
          //Dans le cas d'un mouvement distance on calcule la distance parcourue pour repartir
          //avec une consigne adapte
          DistanceParcourue=sqrt((x_pos-x_old)^2+(y_pos-y_old)^2);
          local_Tempo=0;
          during :
          local_Tempo++;
          state DETECT_OBSTACLE/
            entry :
            local_Tempo = 0;
            Mouvement_ArretBrutal(); // Arrête tout pendant un instant
          state DETECT_OBSTACLE1/
            entry :
            ConsigneVitesseAngle = 3; // [rad/sec]
            ConsigneVitesseDistance = 40; //[cm/sec]
            EvitementEnCours = 0;
          (default) -> DETECT_OBSTACLE
          DETECT_OBSTACLE -> DETECT_OBSTACLE1 : [local_Tempo > (2/Te)]
        STRATEGIE1 -> EVITEMENT : [(isObstacle==1) && (inhibeObstacle==0)]
        (default) -> STRATEGIE1
        EVITEMENT -> STRATEGIE1 : [(EvitementEnCours==0)]
      state CLOCK [parallel]
        during : DureeMatch++
        settings: executionOrder=1
    (default) -> ATTENTE_TIRETTE
    MATCH -> FIN_MATCH : [(DureeMatch > (300/Te)) || (finHomologation==1)]
    ATTENTE_TIRETTE -> MATCH : [Tirette != 0]
  state ret = isFinMouvement(timeout) [function]
    (junction 101) -> (junction 102) : { ret = (CompteurTimeoutMvt > timeout) || (isFrontMontantConvergence(ConvergenceMvt));}
    (default) -> (junction 101) : { CompteurTimeoutMvt++}
  state ret = isFinDetectionObstacle_AV [function]
    (default) -> (junction 108) : { ret =  (((ObstacleAVD==0) && (ObstacleAVG==0) && (STT==1)) || (finObstacle_01==1));}
  state FONCTIONS_GLOBALES_DEPLACEMENT_ROBOT [parallel]
    settings: executionOrder=2
  state Mouvement_Manuel(motG, motD) [function]
    (default) -> (junction 104) : {  DdeMvtManuel = DdeMvtManuel+1;...
        |    CommandeManuelleG = motG;...
        |    CommandeManuelleD = motD;...
        | }
  state FONCTIONS_GLOBALES_COMMANDE_LEDS [parallel]
    settings: executionOrder=5
  state FONCTIONS_GLOBALES_DETECTION_OBSTACLES [parallel]
    settings: executionOrder=4
  state setPWM(idMoteur,pwm) [function]
    (default) -> (junction 115) : {  CommandeMoteur[idMoteur-1] = pwm;
        |  }
  state ret = isDetectionObstacle_AV [function]
    (default) -> (junction 109) : { ret = (ObstacleAVD || ObstacleAVG) && (AutoriseDetectionObstacle_AV != 0) ;}
  state FONCTIONS_GLOBALES_COMMANDE_SERVOS_MOTEURS [parallel]
    settings: executionOrder=3
  state Mouvement_DistanceAngle(dist, teta_rad) [function]
    (default) -> (junction 103) : {  DdeMvtDistanceAngle++;...
        |    ConsigneDistance = dist;...
        |    ConsigneTeta = teta_rad;...
        |    % Modulo de l'angle fait dans le StrategieMatlab.c
        |    CompteurTimeoutMvt = 0;...
        | }
  state Mouvement_XYTeta(x, y,teta_rad) [function]
    (default) -> (junction 114) : {  DdeMvtXYTeta++;...
        |    ConsigneX = x;...
        |    ConsigneY = y;...
        |    ConsigneTeta=teta_rad;...
        |    CompteurTimeoutMvt = 0;...
        | }
  state out_FrontConvergence  = isFrontMontantConvergence(ConvergenceMouvement) [function]
  state out_FrontMvtBloque  = isFrontMontantMvtBloque(ConvergenceMouvement) [function]
  state Mouvement_Angle(teta_rad) [function]
    (default) -> (junction 105) : {  DdeMvtDistanceAngle++;...
        |    ConsigneDistance = 0;...
        |    ConsigneTeta = teta_rad;...
        |    CompteurTimeoutMvt = 0;...
        | }
  state Mouvement_Distance(dist) [function]
    (default) -> (junction 106) : {  DdeMvtDistanceAngle++;...
        |    ConsigneDistance = dist;...
        |    % ConsigneTeta reste inchangé.
        |    CompteurTimeoutMvt = 0;...
        | }
  state CommandeLEDS_RVBO(R, V, B, O) [function]
    (default) -> (junction 107) : {   EtatLed1 = R;...
        |     EtatLed2 = V;...
        |     EtatLed3 = B;...
        |     EtatLed4 = O;...
        | }
  state setDetectionObstacle_AVAR(AV, AR) [function]
    (default) -> (junction 119) : {  AutoriseDetectionObstacle_AV = AV;...
        |    AutoriseDetectionObstacle_AR = AR;
        | }
  state FONCTIONS_GLOBALES_DIVERS [parallel]
    settings: executionOrder=6
  state Mouvement_XY(x, y) [function]
    (default) -> (junction 110) : {  DdeMvtXY++;...
        |    ConsigneX = x;...
        |    ConsigneY = y;...
        |    CompteurTimeoutMvt = 0;...
        | }
  state CommandeLEDS_ARAV(R, V) [function]
    (default) -> (junction 118) : {   %Arrière
        |     EtatLed1 = R;...
        |     %Avant
        |     EtatLed2 = V;
        | }
  state ActiveDetectionObstacle_AV [function]
    (default) -> (junction 130) : {   AutoriseDetectionObstacle_AV =1;
        | }
  state ActiveDetectionObstacle_AR [function]
    (default) -> (junction 127) : {   AutoriseDetectionObstacle_AR = 1;
        | }
  state ret = isDetectionObstacle_AR [function]
    (default) -> (junction 123) : { ret = (ObstacleARG) && (AutoriseDetectionObstacle_AR != 0) ;}
  state RecalagePosition_XYTeta(x, y, teta) [function]
    (default) -> (junction 125) : {  DdeRecalagePosition++;...
        |    ConsigneX = x;...
        |    ConsigneY = y;...
        |    ConsigneTeta = teta
        | }
  state InhibeDetectionObstacle_AV [function]
    (default) -> (junction 122) : {   AutoriseDetectionObstacle_AV = 0;
        | }
  state ret = isFinMouvementRapide(timeout) [function]
    (default) -> (junction 129) : { CompteurTimeoutMvt++}
    (junction 129) -> (junction 113) : { ret = (CompteurTimeoutMvt > timeout) || (isFrontMontantConvergence(ConvergenceMvt_Rapide));}
  state setServo(idServo,pos) [function]
    (default) -> (junction 117) : {  CommandeServo[idServo-1] = pos;
        |  }
  state setServoSpeed(idServo,vit) [function]
    (default) -> (junction 112) : {  SpeedServo[idServo-1] = vit;
        |  }
  state InhibeDetectionObstacle_AR [function]
    (default) -> (junction 100) : {   AutoriseDetectionObstacle_AR = 0;
        | }
  state ret = isMouvementBloque [function]
    (default) -> (junction 126) : { ret =(isFrontMontantMvtBloque(ConvergenceMvt));}
  state ret = isFinDetectionObstacle_AR [function]
    (default) -> (junction 124) : { ret =  (((ObstacleARG==0) && (STT==1)) || (finObstacle_02==1));}
  state Mouvement_DistanceVitesse(dist, vitesse) [function]
    (default) -> (junction 120) : {  DdeMvtDistanceAngle++;...
        |    ConsigneDistance = dist;...
        |    ConsigneVitesseDistance = vitesse;...
        |    % ConsigneTeta reste inchangé.
        |    CompteurTimeoutMvt = 0;...
        | }
  state Mouvement_AngleVitesse(teta_rad, vitesse) [function]
    (default) -> (junction 121) : {  DdeMvtDistanceAngle++;...
        |    ConsigneDistance = 0;...
        |    ConsigneTeta = teta_rad;...
        |    ConsigneVitesseAngle = vitesse;...
        |    CompteurTimeoutMvt = 0;...
        | }
  state FONCTIONS_RECalAGE_POSITION [parallel]
    settings: executionOrder=7
  state Mouvement_ArretBrutal [function]
    (default) -> (junction 131) : { ConsigneVitesseDistance=0;...
        | ConsigneVitesseAngle=0;}
  state setPosition(x, y,teta_rad) [function]
    (default) -> (junction 132) : {  DdeRecalagePosition[0]++;...
        |    DdeRecalagePosition[1] = x;...
        |    DdeRecalagePosition[2] = y;...
        |    DdeRecalagePosition[3] = teta_rad;...
        |    CompteurTimeoutMvt = 0;...
        | }
  state setServoRelache(idServo,tps) [function]
    (default) -> (junction 133) : {  RelacheServo[idServo-1] = (tps*1000);
        |  }
  data: ret function_output double; timeout function_input double; ret function_output double; motG function_input double; motD function_input double; idMoteur function_input double; pwm function_input double; ret function_output double; dist function_input double; teta_rad function_input double; x function_input double; y function_input double; teta_rad function_input double; out_FrontConvergence function_output double; ConvergenceMouvement function_input double; out_FrontMvtBloque function_output double; ConvergenceMouvement function_input double; teta_rad function_input double; dist function_input double; R function_input double; V function_input double; B function_input double; O function_input double; AV function_input double; AR function_input double; x function_input double; y function_input double; R function_input double; V function_input double; ret function_output double; x function_input double; y function_input double; teta function_input double; ret function_output double; timeout function_input double; idServo function_input double; pos function_input double; idServo function_input double; vit function_input double; ret function_output double; ret function_output double; dist function_input double; vitesse function_input double; teta_rad function_input double; vitesse function_input double; x function_input double; y function_input double; teta_rad function_input double; idServo function_input double; tps function_input double; Tirette input double; x_pos input double; y_pos input double; teta_pos input double; ConvergenceMvt input double; CouleurEquipe input double; ObstacleAVG input double; ObstacleAVD input double; ObstacleARG input double; ObstacleARD input double; Temps_absolu input double; AngleVersObjet input double; DistanceVersObjet input double; ConsigneX output double; ConsigneY output double; DdeMvtXY output double; ConsigneTeta output double; ConsigneVitesseAngle output double; ConsigneDistance output double; ConsigneVitesseDistance output double; DdeMvtDistanceAngle output double; CommandeManuelleG output double; CommandeManuelleD output double; DdeMvtManuel output double; DureeMatch local double; Te parameter double; EtatLed1 output double; EtatLed2 output double; EtatLed3 output double; EtatLed4 output double; CouleurEquipe_memo local double; EQUIPE_JAUNE parameter double; CompteurTimeoutMvt local double; AutoriseDetectionObstacle_AV local double; Flag_fin_accostage local double; TetaPos local double; Flag_Fin_Accostage local double; FinMouvementPredefini local double; TempoStabiliseCamera local double; DistanceVersPalet_memo local double; TempoCourante local double; DdeRecalagePosition output double size=4 =0; invMouv local double; TempoCam local double; finHomologation local double; finObstacle_01 local double; PI parameter double; Tempo local double; ConsigneAngle local double; index local double; STT parameter int8; IndexFixed local double; TempoInit local double; JUST_HOMOLO parameter int8; TempoMot local double; ObstacleDetecte local double; TempoImage local double; theta_offset local double; x_offset local double; y_offset local double; N local double; DemandeTestActionneurs input uint8; Etat_Actionneur local double size=[1 10] =[0 0 0 0 0 0 0 0 0 0]; test_actionneurs_en_cours local double; EQUIPE_VERTE parameter double; SERVO_CENTREUR_D_OUVERT parameter double; SERVO_CENTREUR_G_FERME parameter double; SERVO_PINCE_G_FERME parameter double; SERVO_CENTREUR_G_OUVERT parameter double; SERVO_PINCE_D_FERME parameter double; TempoTestActionneurs local double; MAX_SPEED_SERVOS parameter double; TempoTestLED local double; AutoriseDetectionObstacle_AR local double; finObstacle_02 local double; SERVO_PINCE_D_OUVERT parameter double; SERVO_PINCE_G_OUVERT parameter double; besoinInfosCam local double; ElementPiege_AV local double; ElementPiege_AR local double; TempoBO local double; AntiRebond local double; CompteurErreurCapteur local double; CompteurPerteLigne local double; TempoMouvementSuiviLigne local double; EvitementEnCours local double; x_pos_objectif local double; y_pos_objectif local double; RecalageBordureEnCours local double; SERVO_CENTREUR_D_FERME parameter double; DistanceParcourue local double; x_old local double; x_temp local double; y_old local double; y_temp local double; cmptServos local double; IncEtape local double; DistanceParcourue2 local double; x_old2 local double; y_old2 local double; FinCourseAscenseur input uint8; ResetCodeurAscenseur output double =0; ResetCodeurBarillet output double =0; Ascenseur_pos input double; FinCourseBarillet input uint8; Barillet_pos input double; DdeMvtXYTeta output double; ConvergenceMvt_Rapide input double; KMAR_POSITION_HAUT parameter double; KMAR_POSITION_AU_DESSUS_SPOT_AVEC_SPOT parameter double; KMAR_POSITION_SPOT_BAS parameter double; KMAR_POSITION_AU_DESSUS_SPOT_SANS_SPOT parameter double; isDepression input uint8; MODE_XYTETA parameter int8; isObstacle input uint8; local_Tempo local double; isButeeAscenseur local double; local_Tempo_Ascenseur local double; inhibeObstacle local double; FinCourseHauteAscenseur input uint8; DEBUG_TORCHE parameter double; CommandeMoteur output double size=8 =0; MOTEUR_SOUFFLEUR parameter double; CommandeServo output double size=20 =0; SpeedServo output double size=20; SERVO_PINCE_D parameter double; SERVO_PINCE_G parameter double; MOTEUR_ASCENSEUR parameter double; MOTEUR_DISTRIBUTEUR parameter double; MOTEUR_NON_DEFINI parameter double; SERVO_CENTREUR_D parameter double; SERVO_CENTREUR_G parameter double; KMAR_POSITION_DEPART parameter double; RelacheServo output double size=20; SERVO_RECOLTEURS parameter double; SERVO_RECOLTEURS_FERME parameter double; SERVO_RECOLTEURS_OUVERT parameter double; SERVO_PINCE_D_ENTRE_OUVERT parameter double; SERVO_PINCE_G_ENTRE_OUVERT parameter double
